simulink model "sensor_reading"  (R2024a)
settings: Solver=VariableStepAuto  StartTime=0.0  StopTime=inf  MinStep=1e-2  RelTol=1e-3
libraries: read x2, uavutilslib x1, init x1
settings Model: Creator=adriaeik  LastModifiedBy=adriaeik

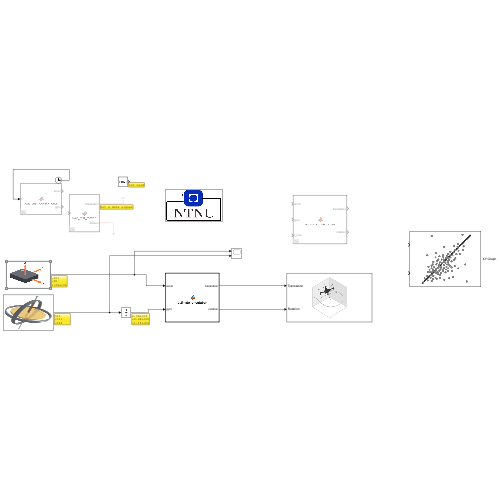
[thumbnail: Simulink's stored preview of the top-level diagram]
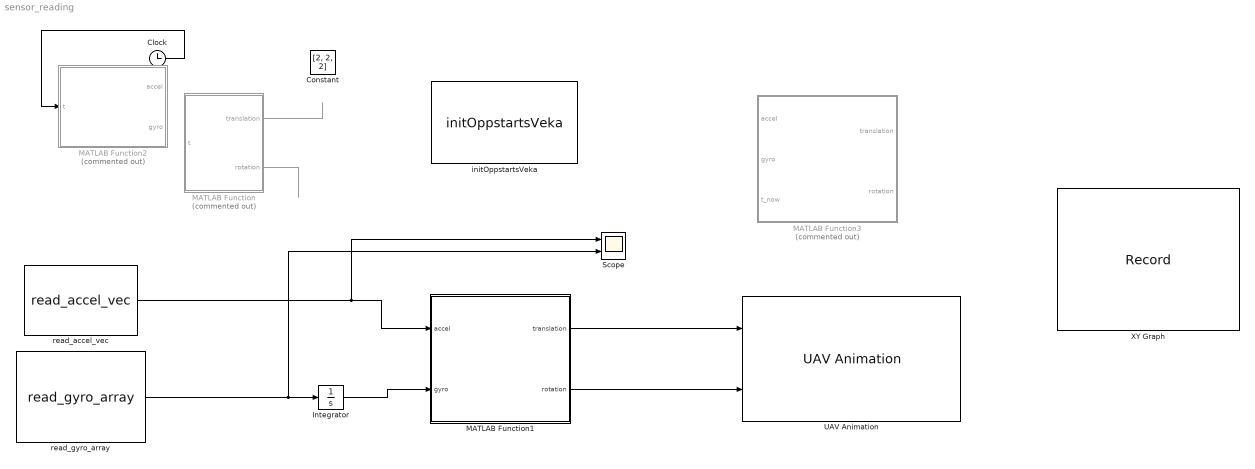
== system sensor_reading ==
  Clock : Clock
  Constant : Constant  Value=[2, 2, 2]
  Integrator : Integrator
  MATLAB Function : MATLAB Function  Commented=on  TreatAsAtomicUnit=on
  MATLAB Function1 : MATLAB Function  TreatAsAtomicUnit=on
  MATLAB Function2 : MATLAB Function  Commented=on  TreatAsAtomicUnit=on
  MATLAB Function3 : MATLAB Function  Commented=on  TreatAsAtomicUnit=on
  Scope : Scope  NumInputPorts=2
  UAV Animation : uavutilslib/UAV Animation  UAVType=Multirotor  UAVSize=1  InertialZDirection=Down  SampleTime=0.1
  XY Graph : Record  FileSettingsInternal="{\"entries\":[{\"content\":{\"excelSettings\":{\"content\":{},\"type\":\"Streamout.ExcelSettings\"}},\"type\":\"Streamout.FileSettingStorage\",\"uuid\":\"\"}],\"packageUris\":[\"http:\\/\\/schema.mathworks.com\\/mf0\\/streamout_blocks\\/R2020a\"],\"version\":\"1.0\"}"  Layout=[1 1]  SignalsInternal="{\"entries\":[{\"content\":{\"signals\":[{\"content\":{\"blockPath\":[],\"dimensions\":[1],\"domain\":\"\",\"lineColor\":\"#a2142f\",\"plots\":[ 1 ],\"port\":1,\"sid\":[\"\"],\"signalID\":1},\"type\":\"RecordBlkView.Signal\",\"uuid\":\"\"},{\"content\":{\"blockPath\":[],\"dimensions\":[1],\"domain\":\"\",\"lineColor\":\"#139fff\",\"plots\":[ 1 ],\"port\":2,\"sid\":[\"\"],\"signalID\":2},\"type\":\"RecordBlkView.Signal\",\"uuid\":\"\"}]},\"type\":\"RecordBlkView.InputSignals\",\"uuid\":\"\"}],\"packageUris\":[\"http:\\/\\/schema.mathworks.com\\/mf0\\/streamout_blocks\\/R2020a\"],\"version\":\"1.0\"}"  VisualizationBindings="{\"xyplotplugin\":{\"info\":[{\"series\":[{\"bindingParametersList\":[{\"parameter\":\"X-Axis\",\"signalID\":1,\"signalName\":\"XY Graph:1\"},{\"parameter\":\"Y-Axis\",\"signalID\":2,\"signalName\":\"XY Graph:2\"}],\"seriesID\":0}],\"subplotID\":1}]}}"  CompatibilityTag=XY
  initOppstartsVeka : init/initOppstartsVeka  carID=14
  read_accel_vec : read/read_accel_vec
  read_gyro_array : read/read_gyro_array
  wires:
  MATLAB Function/1(translation) -> ?
  MATLAB Function/2(rotation) -> ?
  Clock/1 -> MATLAB Function2/1(t)
  MATLAB Function1/1(translation) -> UAV Animation/1
  MATLAB Function1/2(rotation) -> UAV Animation/2
  Integrator/1 -> MATLAB Function1/2(gyro)
  read_accel_vec/1 -> Scope/1, MATLAB Function1/1(accel)
  read_gyro_array/1 -> Scope/2, Integrator/1

== matlab function sensor_reading/MATLAB Function1 ==
  settings: updateMethod=DISCRETE  sampleTime=0.1
  data: accel input; translation output; rotation output; gyro input
function [translation, rotation] = estimate_orientation(accel, gyro)
%#codegen

% accel, gyro: [3x1] vektorar. gyro(3) er ferdig integrert yaw
% Output: 
%   translation: [3x1] vektor
%   rotation:    [4x1] quaternion

% Sørg for riktig format
accel = accel(:);
gyro = gyro(:);

% Konverter yaw frå grader til radianar om nødvendig
yaw = deg2rad(gyro(3));  % kommenter vekk dersom yaw alt er i rad

% Normaliser akselerometer
accel = accel / norm(accel);

% Persistent for filtering
persistent last_pitch last_roll last_yaw
if isempty(last_pitch)
    last_pitch = 0; last_roll = 0; last_yaw = 0;
end

% Estimer pitch og roll frå akselerometer
raw_pitch = atan2(accel(1), sqrt(accel(2)^2 + accel(3)^2));
raw_roll  = atan2(-accel(2), accel(3));

% Lavpassfilter
alpha = 0.95;
pitch = alpha * last_pitch + (1-alpha) * raw_pitch;
roll  = alpha * last_roll  + (1-alpha) * raw_roll;
yaw   = alpha * last_yaw   + (1-alpha) * yaw;

last_pitch = pitch;
last_roll  = roll;
last_yaw   = yaw;

% Konverter Euler-vinklar til quaternion
q = eul2quat([yaw, pitch, roll]);  % rekkefølge: [yaw, pitch, roll]
rotation = reshape(q, [4,1]);      % UAV Animation krev [4x1]

% Stilleståande posisjon
translation = [0; 0; 0];
end

== matlab function sensor_reading/MATLAB Function ==
  data: t input; translation output; rotation output
function [translation, rotation] = uav_test_motion(t)
%#codegen

% Simulert posisjon (sirkel)
x = 5 * cos(0.2 * t);
y = 5 * sin(0.2 * t);
z = 0.5 * sin(0.1 * t);

translation = [x; y; z];

% Euler-vinklar (i radianar)
roll  = 0.2 * sin(0.3 * t);
pitch = 0.2 * cos(0.4 * t);
yaw   = 0.5 * t;

% Konverter Euler → Quaternion [w, x, y, z]
rotation = eul2quat([yaw, pitch, roll]);  % Merk rekkefølge!
end

== matlab function sensor_reading/MATLAB Function2 ==
  data: t input; accel output; gyro output
function [accel, gyro] = simulate_sensor_data(t)
%#codegen

% Parametrar for "rørsle"
yaw_rate   = 0.3 * cos(0.5 * t);    % rad/s, varierande rotasjon rundt Z
pitch_angle = 0.2 * sin(0.3 * t);   % rad
roll_angle  = 0.1 * cos(0.2 * t);   % rad

% Gyro: målte rotasjonshastigheiter
gyro_x = 0;                      % Lite rotasjon i X
gyro_y = 0;                      % Lite rotasjon i Y
gyro_z = yaw_rate;              % Endring i yaw

gyro = [gyro_x, gyro_y, gyro_z];

% Akselerometer: måler tyngdekraft retta mot bakken + bevegelse
% Vi bruker pitch og roll til å berekne tilsynelatande akselerasjon
g = 9.81;

accel_x = g * sin(pitch_angle);
accel_y = -g * sin(roll_angle) * cos(pitch_angle);
accel_z = g * cos(pitch_angle) * cos(roll_angle);

accel = [accel_x, accel_y, accel_z];
end

== matlab function sensor_reading/MATLAB Function3 ==
  data: accel input; translation output; rotation output; gyro input; t_now input
function [translation, rotation] = estimate_orientation(accel, gyro, t_now)
%#codegen

% accel, gyro: [3x1] vektorar
% t_now: tid i sekund (frå Clock)

% Sørg for riktig format
accel = accel(:);
gyro = gyro(:);

% Persistente variablar
persistent yaw t_prev
if isempty(t_prev)
    t_prev = t_now;
    yaw = 0;
end

% Berekn tidssteg
dt = t_now - t_prev;
t_prev = t_now;

% Estimer pitch og roll frå akselerometer
pitch = atan2(accel(1), sqrt(accel(2)^2 + accel(3)^2));
roll  = atan2(-accel(2), accel(3));

% Integrer yaw frå gyro
yaw = yaw + gyro(3) * dt;

% Konverter Euler-vinklar til quaternion
q = eul2quat([yaw, pitch, roll]);  % merk: rekkefølge [yaw, pitch, roll]
rotation = reshape(q, [4,1]);      % tving til [4x1] for UAV Animation

% Stilleståande posisjon
translation = [0; 0; 0];
end
